simulink model "EffectuatorIntegratedWithDemonstrator"  (R2020a)
settings: Solver=FixedStepDiscrete  StartTime=0.0  StopTime=inf  FixedStep=Ts  RelTol=1e-3
InitFcn:
  | %% Verwende vordefinierte Setpoints (Kreis mit Z-Komponente)
  | 
  | % Config
  | numCircles = 3;
  | scale=6;
  | %Versuch symmetrische Setpunkte zu setzen
  | pointsPerCircle =scale*(4+3*numCircles)+2;
  | 
  | r = 50;
  | m_x = r;
  | m_y = r;
  | 
  | % //
  | s = linspace(0,2*pi,pointsPerCircle);
  | 
  | setPoints_x = [];
  | setPoints_y = [];
  | 
  | for ii=1:numCircles
  | 
  | setPoints_x = [setPoints_x (-cos(s(1:floor(pointsPerCircle / 2))).*r + m_x + 2*r*(ii-1))]; %#ok<AGROW>
  | setPoints_y = [setPoints_y (sin(s).*r+m_y)]; %#ok<AGROW>pointsPerCircle / 2
  | 
  | end
  | 
  | setPoints_x = [setPoints_x flip(setPoints_x(1:end))];
  | 
  | % Loeschen doppelter y-Werte (Kreisuebergang)
  | setPoints_x(pointsPerCircle .* [1:numCircles]) = [];
  | setPoints_y(pointsPerCircle .* [1:numCircles]) = [];
  | 
  | % setPoints_x= [linspace(0,setPoints_x(19),19) setPoints_x(20:end)];
  | % setPoints_y= [linspace(0,setPoints_y(19),19) setPoints_y(20:end)];
  | 
  | % Array Elemente verschieben
  | % setPoints_x = circshift(setPoints_x,-pointsPerCircle/4,2);
  | % setPoints_y = circshift(setPoints_y,-pointsPerCircle/4,2);
  | 
  | z = zeros(1,size(setPoints_x,2));
  | z_x = -5:5;
  | z_y = -z_x.^2 + 25;
  | z_idx = 90;
  | z_idx2 = 210;
  | z(z_idx:z_idx+length(z_x)-1) = z_y;
  | z(z_idx2:z_idx2+length(z_x)-1) = z_y;
  | % z = [z_y z];
  | setPoints_z = z;
  | 
  | % setPoints_x = [zeros(1,length(z_y)) setPoints_x];
  | % setPoints_y = [setPoints_y(1,1)*ones(1,length(z_y)) setPoints_y];
  | 
  | % Umrechnung der Einheiten für Demonstrator
  | % setPoints_x = setPoints_x ./ 1000;
  | % setPoints_y = setPoints_y ./ 1000;
  | % setPoints_z = setPoints_z ./ 1000;
  | 
  | 
  | %{
  | plot(setPoints_x,setPoints_y);
  | fig = figure;
  | ... (+13 lines)
StartFcn:
  | close all;
model workspace (MAT data in the model file):
  MvmtPerfEval_collectVal : Simulink.Parameter (value not decoded)
  MvmtPerfEval_sendOwnVal : Simulink.Parameter (value not decoded)
  PerfEval_numTicks_enable : Simulink.Parameter (value not decoded)
  Segmentregler_I_Gain : Simulink.Parameter (value not decoded)
  Segmentregler_P_Gain : Simulink.Parameter (value not decoded)
  Segmentregler_minVel_enable : Simulink.Parameter (value not decoded)
  Segmentregler_numTicks_enable : Simulink.Parameter (value not decoded)
  Ts : Simulink.Parameter (value not decoded)
  maxPos_x : Simulink.Parameter (value not decoded)
  maxPos_y : Simulink.Parameter (value not decoded)
  maxPos_z : Simulink.Parameter (value not decoded)
  maxVectorLengths : Simulink.Parameter (value not decoded)
  minAllowedVelSaturation : Simulink.Parameter (value not decoded)
  numAxes : Simulink.Parameter (value not decoded)
symbols that are objects in the model workspace (value not decoded): maxPos_x, maxPos_y, maxPos_z, minAllowedVelSaturation, MvmtPerfEval_collectVal, MvmtPerfEval_sendOwnVal, numAxes, PerfEval_numTicks_enable, Segmentregler_I_Gain, Segmentregler_minVel_enable, Segmentregler_numTicks_enable, Segmentregler_P_Gain, Ts
undefined symbols (not defined in the file or in its folder): DiscIntNeverNeededParam, VelOverride
libraries: simulink x20, vrlib x5, sldrtlib x2, xpcrtudplib x2, dspnetwork x2, ptplib x1, etargetslib x1, xpcutilitieslib x1
(part 5 of 5)

== stateflow chart EffectuatorIntegratedWithDemonstrator/MASTER ==
  state funcs [group]
  state Dispatcher [parallel]
    settings: executionOrder=1
    state Idle
    state Registriere_Achse
      entry: num_registeredAxes = ...
      num_registeredAxes + 1;
    state Erhalte_Koordinationsvektor
      entry:
      num_collectedCVectors = ...
      num_collectedCVectors + 1;
      cVectors = [cVectors; cVector_exchange];
      FLAG_canSend_cVector = 1;
    state Distribute_Coordination_Info
      entry:
      FLAG_cVectors_complete = 1;
    state Registriere_Achsen_bereit
      entry:
      num_readyAxes = num_readyAxes + 1;
      if(num_readyAxes == num_registeredAxes)
      FLAG_allAxesReady = 1;
      messageToEffectuator=2;
      end
    state DONE
      entry:
      num_doneAxes = num_doneAxes + 1;
      if num_doneAxes == num_registeredAxes
      FLAG_stopSim = 1;
      end
    state Movement_Performance_Evaluation
      entry:
      segmentDone=segmentDone+1;
      if (segmentDone==num_registeredAxes)
      canStartNewSegment=1;
      segmentDone=0;
      else
      canStartNewSegment=0;
      end
      while receive(MvmtPerfCoeff)
      if MvmtPerfCoeff.data > MvmtPerf
      MvmtPerf = MvmtPerfCoeff.data;
      end
      if MvmtPerfCoeff.data == -1
      MvmtPerf = 1;
      end
      discard(MvmtPerfCoeff);
      end
    (default) -> Idle
    Idle -> Registriere_Achse [order 1] : registerAxis
    Registriere_Achse -> Idle
    Idle -> Erhalte_Koordinationsvektor [order 2] : cVector_sent
    Erhalte_Koordinationsvektor -> Idle
    Idle -> Distribute_Coordination_Info [order 3] : [num_collectedCVectors==...
        | num_registeredAxes && ...
        | FLAG_cVectors_complete == 0]
    Distribute_Coordination_Info -> Idle
    Idle -> Registriere_Achsen_bereit [order 4] : axis_ready
    Registriere_Achsen_bereit -> Idle
    Idle -> Dispatcher.DONE [order 5] : axis_done
    Dispatcher.DONE -> Idle
    Idle -> Movement_Performance_Evaluation [order 6] : MvmtPerfCoeff
    Movement_Performance_Evaluation -> Idle
  state Axis_X [parallel]
    settings: executionOrder=2
    state Start_Idle
      entry:
      registerAxis.data = true;
      send(registerAxis)
    state Hermite_Interpolation
      entry:
      if FLAG_doAkima == 1
      iP = funcs.DS_hermIntp(setP,setP_dist);
      else
      iP = setP;
      end
    state Koordinationsvektor
      entry:
      cVector_init = funcs.DS_gen_Cvector_init...
      (iP,PAR_isAxis,PAR_maxVel);
    state Koordinationsvektor_austauschen
      during:
      if FLAG_canSend_cVector == 1
      cVector_exchange = cVector_init;
      FLAG_canSend_cVector = 0;
      send(cVector_sent);
      axisHasSentCVector = 1;
      end
      Axis_X.Koordinationsvektor_austauschen -> Axis_X.Koordinationsvektor_austauschen [order 1]
    state Wait_for_cVectors
    state Find_Consensus
      entry: execVec = funcs.DS_find_Consensus(iP,cVectors,...
      PAR_execIteratorStepSize,PAR_isAxis);
      send(axis_ready);
    state Start_run
      entry:
      RUN_idx = 0;
      RUN_startPos(1,PAR_isAxis) = setP(PAR_isAxis,1);
      RUN_num_steps = size(execVec,2);
      state Send_command
        entry:
        RUN_idx = RUN_idx + 1;
        currCVector = cVectors(:,RUN_idx)' ./ VelOverride';
        currCVal = max(currCVector);
        currOverrideAdaptationFactor = execVec(3,RUN_idx) / currCVal; %individueller neuer Override Faktor für diese Achse
        currStepTimeLength = execVec(3,RUN_idx) / currOverrideAdaptationFactor;
        RUN_pos(1,PAR_isAxis) = execVec(1,RUN_idx);
        RUN_vel(1,PAR_isAxis) = execVec(2,RUN_idx) * currOverrideAdaptationFactor;
        MvmtPerf_accumulatedLagTime = MvmtPerf_accumulatedLagTime + (currStepTimeLength - execVec(3,RUN_idx));
        RUN_time(1,PAR_isAxis) = execVec(4,RUN_idx) + MvmtPerf_accumulatedLagTime; %wird nicht benutzt
        RUN_maxVel(1,PAR_isAxis) = PAR_maxVel;
        RUN_MvmtPerfFeedback(1,PAR_isAxis) = 0; %wird zZt nicht benutzt
      state execute_movement
        state idle
          entry:
          MvmtPerfCoeff.data = -1;
          send(MvmtPerfCoeff);
        state getOwnPerfCoeff [commented out]
          entry:
          MvmtPerfCoeff.data = GET_perfIndicator(PAR_isAxis);
          send(MvmtPerfCoeff);
        state getMutualPerformance [commented out]
          entry:
          MvmtPerf_accumulatedLagTime = MvmtPerf_accumulatedLagTime + (MvmtPerf-1) * currStepTimeLength;
          RUN_MvmtPerfFeedback(1,PAR_isAxis) = (MvmtPerf-1) * currStepTimeLength;
          RUN_vel(1,PAR_isAxis) = execVec(2,RUN_idx) / MvmtPerf;
          currStepTimeLength = currStepTimeLength * MvmtPerf;
        (default) -> Axis_X.Start_run.execute_movement.idle
        Axis_X.Start_run.execute_movement.idle -> Axis_X.Start_run.execute_movement.getOwnPerfCoeff [commented out] : after(currStepTimeLength * MvmtPerfEval_sendOwnVal,sec)
        Axis_X.Start_run.execute_movement.getOwnPerfCoeff -> Axis_X.Start_run.execute_movement.getMutualPerformance [commented out] : after(currStepTimeLength * (MvmtPerfEval_collectVal - MvmtPerfEval_sendOwnVal),sec)
      (default) -> Axis_X.Start_run.Send_command
      (junction 638) -> Axis_X.Start_run.Send_command [order 2]
      Axis_X.Start_run.Send_command -> Axis_X.Start_run.execute_movement
      (junction 1327) -> (junction 638) : [index<=EffSegment(1)]
      Axis_X.Start_run.execute_movement -> (junction 1327) : after(currStepTimeLength,sec)
    state DONE
      entry:
      send(axis_done);
    (default) -> Axis_X.Start_Idle
    Axis_X.Start_Idle -> Axis_X.Hermite_Interpolation
    Axis_X.Hermite_Interpolation -> Axis_X.Koordinationsvektor
    Axis_X.Koordinationsvektor -> Axis_X.Koordinationsvektor_austauschen
    Axis_X.Koordinationsvektor_austauschen -> Axis_X.Wait_for_cVectors [order 1] : [axisHasSentCVector == 1]
    Axis_X.Wait_for_cVectors -> Axis_X.Find_Consensus : [FLAG_cVectors_complete == 1]
    Axis_X.Find_Consensus -> Axis_X.Start_run : [FLAG_allAxesReady == 1]
    (junction 638) -> Axis_X.DONE [order 1] : [RUN_idx == RUN_num_steps]
  state Axis_Y [parallel]
    settings: executionOrder=3
    state Start_Idle
      entry:
      registerAxis.data = true;
      send(registerAxis)
    state Hermite_Interpolation
      entry:
      if FLAG_doAkima == 1
      iP = funcs.DS_hermIntp(setP,setP_dist);
      else
      iP = setP;
      end
    state Koordinationsvektor
      entry:
      cVector_init = funcs.DS_gen_Cvector_init...
      (iP,PAR_isAxis,PAR_maxVel);
    state Koordinationsvektor_austauschen
      during:
      if FLAG_canSend_cVector == 1
      cVector_exchange = cVector_init;
      FLAG_canSend_cVector = 0;
      send(cVector_sent);
      axisHasSentCVector = 1;
      end
      Axis_Y.Koordinationsvektor_austauschen -> Axis_Y.Koordinationsvektor_austauschen [order 1]
    state Wait_for_cVectors
    state Find_Consensus
      entry: execVec = funcs.DS_find_Consensus(iP,cVectors,...
      PAR_execIteratorStepSize,PAR_isAxis);
      send(axis_ready);
    state Start_run
      entry:
      RUN_idx = 0;
      RUN_startPos(1,PAR_isAxis) = setP(PAR_isAxis,1);
      RUN_num_steps = size(execVec,2);
      state Send_command
        entry:
        RUN_idx = RUN_idx + 1;
        currCVector = cVectors(:,RUN_idx)' ./ VelOverride';
        currCVal = max(currCVector);
        currOverrideAdaptationFactor = execVec(3,RUN_idx) / currCVal; %individueller neuer Override Faktor für diese Achse
        currStepTimeLength = execVec(3,RUN_idx) / currOverrideAdaptationFactor;
        RUN_pos(1,PAR_isAxis) = execVec(1,RUN_idx);
        RUN_vel(1,PAR_isAxis) = execVec(2,RUN_idx) * currOverrideAdaptationFactor;
        MvmtPerf_accumulatedLagTime = MvmtPerf_accumulatedLagTime + (currStepTimeLength - execVec(3,RUN_idx));
        RUN_time(1,PAR_isAxis) = execVec(4,RUN_idx) + MvmtPerf_accumulatedLagTime; %wird nicht benutzt
        RUN_maxVel(1,PAR_isAxis) = PAR_maxVel;
        RUN_MvmtPerfFeedback(1,PAR_isAxis) = 0; %wird zZt nicht benutzt
      state execute_movement
        state idle
          entry:
          MvmtPerfCoeff.data = -1;
          send(MvmtPerfCoeff);
          index=RUN_idx;
        state getOwnPerfCoeff [commented out]
          entry:
          MvmtPerfCoeff.data = GET_perfIndicator(PAR_isAxis);
          send(MvmtPerfCoeff);
        state getMutualPerformance [commented out]
          entry:
          MvmtPerf_accumulatedLagTime = MvmtPerf_accumulatedLagTime + (MvmtPerf-1) * currStepTimeLength;
          RUN_MvmtPerfFeedback(1,PAR_isAxis) = (MvmtPerf-1) * currStepTimeLength;
          RUN_vel(1,PAR_isAxis) = execVec(2,RUN_idx) / MvmtPerf;
          currStepTimeLength = currStepTimeLength * MvmtPerf;
        (default) -> Axis_Y.Start_run.execute_movement.idle
        Axis_Y.Start_run.execute_movement.idle -> Axis_Y.Start_run.execute_movement.getOwnPerfCoeff [commented out] : after(currStepTimeLength * MvmtPerfEval_sendOwnVal,sec)
        Axis_Y.Start_run.execute_movement.getOwnPerfCoeff -> Axis_Y.Start_run.execute_movement.getMutualPerformance [commented out] : after(currStepTimeLength * (MvmtPerfEval_collectVal - MvmtPerfEval_sendOwnVal),sec)
      (default) -> Axis_Y.Start_run.Send_command
      (junction 1151) -> Axis_Y.Start_run.Send_command [order 2]
      Axis_Y.Start_run.Send_command -> Axis_Y.Start_run.execute_movement
      (junction 1322) -> (junction 1151) : [index<=EffSegment(1)]
      Axis_Y.Start_run.execute_movement -> (junction 1322) : after(currStepTimeLength,sec)
    state DONE
      entry:
      send(axis_done);
    (default) -> Axis_Y.Start_Idle
    Axis_Y.Start_Idle -> Axis_Y.Hermite_Interpolation
    Axis_Y.Hermite_Interpolation -> Axis_Y.Koordinationsvektor
    Axis_Y.Koordinationsvektor -> Axis_Y.Koordinationsvektor_austauschen
    Axis_Y.Koordinationsvektor_austauschen -> Axis_Y.Wait_for_cVectors [order 1] : [axisHasSentCVector == 1]
    Axis_Y.Wait_for_cVectors -> Axis_Y.Find_Consensus : [FLAG_cVectors_complete == 1]
    Axis_Y.Find_Consensus -> Axis_Y.Start_run : [FLAG_allAxesReady == 1]
    (junction 1151) -> Axis_Y.DONE [order 1] : [RUN_idx == RUN_num_steps]
  state Axis_Z [parallel]
    settings: executionOrder=4
    state Start_Idle
      entry:
      registerAxis.data = true;
      send(registerAxis)
    state Hermite_Interpolation
      entry:
      if FLAG_doAkima == 1
      iP = funcs.DS_hermIntp(setP,setP_dist);
      else
      iP = setP;
      end
    state Koordinationsvektor
      entry:
      cVector_init = funcs.DS_gen_Cvector_init...
      (iP,PAR_isAxis,PAR_maxVel);
    state Koordinationsvektor_austauschen
      during:
      if FLAG_canSend_cVector == 1
      cVector_exchange = cVector_init;
      FLAG_canSend_cVector = 0;
      send(cVector_sent);
      axisHasSentCVector = 1;
      end
      Axis_Z.Koordinationsvektor_austauschen -> Axis_Z.Koordinationsvektor_austauschen [order 1]
    state Wait_for_cVectors
    state Find_Consensus
      entry: execVec = funcs.DS_find_Consensus(iP,cVectors,...
      PAR_execIteratorStepSize,PAR_isAxis);
      send(axis_ready);
    state Start_run
      entry:
      RUN_idx = 0;
      RUN_startPos(1,PAR_isAxis) = setP(PAR_isAxis,1);
      RUN_num_steps = size(execVec,2);
      state Send_command
        entry:
        RUN_idx = RUN_idx + 1;
        currCVector = cVectors(:,RUN_idx)' ./ VelOverride';
        currCVal = max(currCVector);
        currOverrideAdaptationFactor = execVec(3,RUN_idx) / currCVal; %individueller neuer Override Faktor für diese Achse
        currStepTimeLength = execVec(3,RUN_idx) / currOverrideAdaptationFactor;
        RUN_pos(1,PAR_isAxis) = execVec(1,RUN_idx);
        RUN_vel(1,PAR_isAxis) = execVec(2,RUN_idx) * currOverrideAdaptationFactor;
        MvmtPerf_accumulatedLagTime = MvmtPerf_accumulatedLagTime + (currStepTimeLength - execVec(3,RUN_idx));
        RUN_time(1,PAR_isAxis) = execVec(4,RUN_idx) + MvmtPerf_accumulatedLagTime; %wird nicht benutzt
        RUN_maxVel(1,PAR_isAxis) = PAR_maxVel;
        RUN_MvmtPerfFeedback(1,PAR_isAxis) = 0; %wird zZt nicht benutzt
      state execute_movement
        state idle
          entry:
          MvmtPerfCoeff.data = -1;
          send(MvmtPerfCoeff);
        state getOwnPerfCoeff [commented out]
          entry:
          MvmtPerfCoeff.data = GET_perfIndicator(PAR_isAxis);
          send(MvmtPerfCoeff);
        state getMutualPerformance [commented out]
          entry:
          MvmtPerf_accumulatedLagTime = MvmtPerf_accumulatedLagTime + (MvmtPerf-1) * currStepTimeLength;
          RUN_MvmtPerfFeedback(1,PAR_isAxis) = (MvmtPerf-1) * currStepTimeLength;
          RUN_vel(1,PAR_isAxis) = execVec(2,RUN_idx) / MvmtPerf;
          currStepTimeLength = currStepTimeLength * MvmtPerf;
        (default) -> Axis_Z.Start_run.execute_movement.idle
        Axis_Z.Start_run.execute_movement.idle -> Axis_Z.Start_run.execute_movement.getOwnPerfCoeff [commented out] : after(currStepTimeLength * MvmtPerfEval_sendOwnVal,sec)
        Axis_Z.Start_run.execute_movement.getOwnPerfCoeff -> Axis_Z.Start_run.execute_movement.getMutualPerformance [commented out] : after(currStepTimeLength * (MvmtPerfEval_collectVal - MvmtPerfEval_sendOwnVal),sec)
      (default) -> Axis_Z.Start_run.Send_command
      (junction 1195) -> Axis_Z.Start_run.Send_command [order 2]
      Axis_Z.Start_run.Send_command -> Axis_Z.Start_run.execute_movement
      (junction 1320) -> (junction 1195) : [index<=EffSegment(1)]
      Axis_Z.Start_run.execute_movement -> (junction 1320) : after(currStepTimeLength,sec)
    state DONE
      entry:
      send(axis_done);
    (default) -> Axis_Z.Start_Idle
    Axis_Z.Start_Idle -> Axis_Z.Hermite_Interpolation
    Axis_Z.Hermite_Interpolation -> Axis_Z.Koordinationsvektor
    Axis_Z.Koordinationsvektor -> Axis_Z.Koordinationsvektor_austauschen
    Axis_Z.Koordinationsvektor_austauschen -> Axis_Z.Wait_for_cVectors [order 1] : [axisHasSentCVector == 1]
    Axis_Z.Wait_for_cVectors -> Axis_Z.Find_Consensus : [FLAG_cVectors_complete == 1]
    Axis_Z.Find_Consensus -> Axis_Z.Start_run : [FLAG_allAxesReady == 1]
    (junction 1195) -> Axis_Z.DONE [order 1] : [RUN_idx == RUN_num_steps]
  state Axis_X2_Effectuator [parallel]
    settings: executionOrder=5
    state Start_Idle
      entry:
      registerAxis.data = true;
      send(registerAxis)
    state Hermite_Interpolation
      entry:
      if FLAG_doAkima == 1
      iP = funcs.DS_hermIntp(setP,setP_dist);
      else
      iP = setP;
      end
    state Koordinationsvektor
      entry:
      cVector_init = Axis_X2_koordVector;
    state Koordinationsvektor_austauschen
      during:
      if FLAG_canSend_cVector == 1
      cVector_exchange = cVector_init;
      FLAG_canSend_cVector = 0;
      send(cVector_sent);
      axisHasSentCVector = 1;
      messageToEffectuator=1;
      end
      Axis_X2_Effectuator.Koordinationsvektor_austauschen -> Axis_X2_Effectuator.Koordinationsvektor_austauschen [commented out]
    state Wait_for_cVectors
    state Find_Consensus
      entry: execVec =Axis_X2_consusVector;
      send(axis_ready);
    state execute_movement1 [commented out]
      state idle [commented out]
        entry:
        MvmtPerfCoeff.data = -1;
        send(MvmtPerfCoeff);
      state getOwnPerfCoeff [commented out]
        entry:
        MvmtPerfCoeff.data = GET_perfIndicator(PAR_isAxis);
        send(MvmtPerfCoeff);
      state getMutualPerformance [commented out]
        entry:
        MvmtPerf_accumulatedLagTime = MvmtPerf_accumulatedLagTime + (MvmtPerf-1) * currStepTimeLength;
        RUN_MvmtPerfFeedback(1,PAR_isAxis) = (MvmtPerf-1) * currStepTimeLength;
        RUN_vel(1,PAR_isAxis) = execVec(2,RUN_idx) / MvmtPerf;
        currStepTimeLength = currStepTimeLength * MvmtPerf;
      (default) -> Axis_X2_Effectuator.execute_movement1.idle [commented out]
      Axis_X2_Effectuator.execute_movement1.idle -> Axis_X2_Effectuator.execute_movement1.getOwnPerfCoeff [commented out] : after(currStepTimeLength * MvmtPerfEval_sendOwnVal,sec)
      Axis_X2_Effectuator.execute_movement1.getOwnPerfCoeff -> Axis_X2_Effectuator.execute_movement1.getMutualPerformance [commented out] : after(currStepTimeLength * (MvmtPerfEval_collectVal - MvmtPerfEval_sendOwnVal),sec)
    state Start_run [commented out]
      entry:
      RUN_idx = 0;
      RUN_startPos(1,PAR_isAxis) = setP(PAR_isAxis,1);
      RUN_num_steps = size(execVec,2);
      state Send_command [commented out]
        entry:
        RUN_idx = RUN_idx + 1;
        currCVector = cVectors(:,RUN_idx)' ./ VelOverride';
        currCVal = max(currCVector);
        currOverrideAdaptationFactor = execVec(3,RUN_idx) / currCVal; %individueller neuer Override Faktor für diese Achse
        currStepTimeLength = execVec(3,RUN_idx) / currOverrideAdaptationFactor;
        RUN_pos(1,PAR_isAxis) = execVec(1,RUN_idx);
        RUN_vel(1,PAR_isAxis) = execVec(2,RUN_idx) * currOverrideAdaptationFactor;
        MvmtPerf_accumulatedLagTime = MvmtPerf_accumulatedLagTime + (currStepTimeLength - execVec(3,RUN_idx));
        RUN_time(1,PAR_isAxis) = execVec(4,RUN_idx) + MvmtPerf_accumulatedLagTime; %wird nicht benutzt
        RUN_maxVel(1,PAR_isAxis) = PAR_maxVel;
        RUN_MvmtPerfFeedback(1,PAR_isAxis) = 0; %wird zZt nicht benutzt
      state execute_movement [commented out]
        state idle [commented out]
          entry:
          MvmtPerfCoeff.data = -1;
          send(MvmtPerfCoeff);
        state getOwnPerfCoeff [commented out]
          entry:
          MvmtPerfCoeff.data = GET_perfIndicator(PAR_isAxis);
          send(MvmtPerfCoeff);
        state getMutualPerformance [commented out]
          entry:
          MvmtPerf_accumulatedLagTime = MvmtPerf_accumulatedLagTime + (MvmtPerf-1) * currStepTimeLength;
          RUN_MvmtPerfFeedback(1,PAR_isAxis) = (MvmtPerf-1) * currStepTimeLength;
          RUN_vel(1,PAR_isAxis) = execVec(2,RUN_idx) / MvmtPerf;
          currStepTimeLength = currStepTimeLength * MvmtPerf;
        (default) -> Axis_X2_Effectuator.Start_run.execute_movement.idle [commented out]
        Axis_X2_Effectuator.Start_run.execute_movement.idle -> Axis_X2_Effectuator.Start_run.execute_movement.getOwnPerfCoeff [commented out] : after(currStepTimeLength * MvmtPerfEval_sendOwnVal,sec)
        Axis_X2_Effectuator.Start_run.execute_movement.getOwnPerfCoeff -> Axis_X2_Effectuator.Start_run.execute_movement.getMutualPerformance [commented out] : after(currStepTimeLength * (MvmtPerfEval_collectVal - MvmtPerfEval_sendOwnVal),sec)
      (default) -> Axis_X2_Effectuator.Start_run.Send_command [commented out]
      (junction 1244) -> Axis_X2_Effectuator.Start_run.Send_command [commented out]
      Axis_X2_Effectuator.Start_run.Send_command -> Axis_X2_Effectuator.Start_run.execute_movement [commented out]
      Axis_X2_Effectuator.Start_run.execute_movement -> (junction 1244) [commented out] : after(currStepTimeLength,sec)
    state DONE
      entry:
      send(axis_done);
    (default) -> Axis_X2_Effectuator.Start_Idle
    Axis_X2_Effectuator.Start_Idle -> Axis_X2_Effectuator.Hermite_Interpolation
    Axis_X2_Effectuator.Hermite_Interpolation -> Axis_X2_Effectuator.Koordinationsvektor : [messageFromEffectuator==1]
    Axis_X2_Effectuator.Koordinationsvektor -> Axis_X2_Effectuator.Koordinationsvektor_austauschen
    Axis_X2_Effectuator.Koordinationsvektor_austauschen -> Axis_X2_Effectuator.Wait_for_cVectors : [axisHasSentCVector == 1]
    Axis_X2_Effectuator.Wait_for_cVectors -> Axis_X2_Effectuator.Find_Consensus : [FLAG_cVectors_complete == 1&&messageFromEffectuator==2]
    Axis_X2_Effectuator.Find_Consensus -> Axis_X2_Effectuator.DONE : [messageFromEffectuator==4]
  data: inp_data function_input; iPoints function_output; iP_dist function_input; inp_data function_input; whichAxis function_input; cV_init function_output; maxV function_input; iPoints function_input; cVec function_input; execVec function_output; iteratorStep function_input; whichAxis function_input; inp_data function_input; iPoints function_output; iP_dist function_input; num_registeredAxes local =0; num_collectedCVectors local =0; iP local size=[numAxes maxVectorLengths]; cVector_init local size=[1 maxVectorLengths]; PAR_isAxis constant double =1; PAR_maxVel constant double =10; axisHasSentCVector local =0; execVec local size=[4 maxVectorLengths] =1; RUN_idx local double size=1 =0; currStepTimeLength local =0; RUN_num_steps local =0; MvmtPerf_accumulatedLagTime local =0; currCVector local size=[1 numAxes] =zeros(1,numAxes); currCVal local =0; currOverrideAdaptationFactor local =1; isUDP_Agent local =0; iP local size=[numAxes maxVectorLengths]; cVector_init local size=[1 maxVectorLengths]; PAR_isAxis constant double =2; PAR_maxVel constant double =5; axisHasSentCVector local =0; execVec local size=[4 maxVectorLengths] =1; RUN_idx local size=1 =0; currStepTimeLength local =0; RUN_num_steps local =0; MvmtPerf_accumulatedLagTime local =0; currCVector local size=[1 numAxes] =zeros(1,numAxes); currCVal local =0; currOverrideAdaptationFactor local =1; isUDP_Agent local =0; iP local size=[numAxes maxVectorLengths]; cVector_init local size=[1 maxVectorLengths]; PAR_isAxis constant double =3; PAR_maxVel constant double =2; axisHasSentCVector local =0; execVec local size=[4 maxVectorLengths] =1; RUN_idx local size=1 =0; currStepTimeLength local =0; RUN_num_steps local =0; MvmtPerf_accumulatedLagTime local =0; currCVector local size=[1 numAxes] =zeros(1,numAxes); currCVal local =0; currOverrideAdaptationFactor local =1; isUDP_Agent local =0; iP local size=[numAxes maxVectorLengths]; cVector_init local size=[1 maxVectorLengths]; PAR_isAxis constant double =4; PAR_maxVel constant double =5; axisHasSentCVector local =0; execVec local size=[4 maxVectorLengths] =1; RUN_idx local size=1 =0; currStepTimeLength local =0; RUN_num_steps local =0; MvmtPerf_accumulatedLagTime local =0; currCVector local size=[1 numAxes] =zeros(1,numAxes); currCVal local =0; currOverrideAdaptationFactor local =1; isUDP_Agent local =1; setP input; setP_dist input; registerAxis local; FLAG_canSend_cVector local =1; cVector_exchange local size=[1 maxVectorLengths]; cVector_sent local =1; FLAG_cVectors_complete local =0; PAR_execIteratorStepSize constant double =1; axis_ready local =0; num_readyAxes local =0; FLAG_allAxesReady local =0; FLAG_doAkima local =0; axis_done local =0; FLAG_stopSim output =0; RUN_maxVel output size=[1 numAxes] =zeros(1,numAxes); RUN_pos output size=[1 numAxes] =zeros(1,numAxes); RUN_startPos output size=[1 numAxes] =zeros(1,numAxes); RUN_time output size=[1 numAxes] =zeros(1,numAxes); RUN_vel output size=[1 numAxes] =zeros(1,numAxes); MvmtPerfEval_sendOwnVal parameter; GET_perfIndicator data_store_memory; MvmtPerfCoeff local =1; MvmtPerf local =1; RUN_MvmtPerfFeedback output size=[1 numAxes] =zeros(1,numAxes); MvmtPerfEval_collectVal parameter; VelOverride data_store_memory; cVectors output size=[numAxes maxVectorLengths] =0; Axis_X2_koordVector input; Axis_X2_consusVector input; messageFromEffectuator input int32 [..int32(0)]; messageToEffectuator output int32 =int32(0); num_doneAxes output =0; EffSegment input; segmentDone local =0; canStartNewSegment output =0; index output
  events: event local FUNCTION_CALL_EVENT
  function iPoints = DS_hermIntp(inp_data,iP_dist):
    | function iPoints = DS_hermIntp(inp_data,iP_dist)
    |  
    | 
    | euklid_abstand = vecnorm(diff(inp_data,1,2));
    | 
    | laufparam = cumsum(euklid_abstand);
    | laufparam = laufparam / max(laufparam);
    | laufparam = [0 laufparam];
    | 
    | 
    | anzahl_stuetzpunkte = 150;
    | anzahl_dim = size(inp_data,1);
    | iPoints = zeros(anzahl_dim,anzahl_stuetzpunkte);
    | 
    | for i=1:anzahl_dim
    |    
    |     iPoints(i,:) = pchip(laufparam,inp_data(i,:),linspace(0,1,anzahl_stuetzpunkte));
    |     
    | end
    | 
    | end
  function cV_init = DS_gen_Cvector_init(inp_data,whichAxis,maxV):
    | function cV_init = DS_gen_Cvector_init(inp_data,whichAxis,maxV)
    | 
    | safety_margin = 0.2; % max. Geschwindigkeit wird auf 80% der eigentlichen Fähigkeit der Achse festgelegt
    | 
    | wegdaten_raw = inp_data(whichAxis,:);
    | 
    | streckensegmente_raw = diff(wegdaten_raw);
    | 
    | 
    | zeitsegmente_raw = streckensegmente_raw ./ (maxV * (1 - safety_margin));
    | 
    | 
    | cV_init = abs(zeitsegmente_raw);
    | 
    | end
  function execVec = DS_find_Consensus(iPoints,cVec,iteratorStep,whichAxis):
    | function execVec = DS_find_Consensus(iPoints,cVec,iteratorStep,whichAxis)
    | 
    | cVector = max(cVec);
    | 
    | if(iteratorStep > 1)
    |    
    |     if(mod(size(iPoints,2)-1,iteratorStep) == 0)
    |         
    |         array_size = (size(iPoints,2) - 1) / iteratorStep;
    |         iPoints_relevant = zeros(1,array_size);
    |         
    |     else
    |        
    |         array_size = floor((size(iPoints,2) - 1) / iteratorStep) + 1;
    |         iPoints_relevant = zeros(1,array_size);
    |         
    |     end
    |     
    |     
    |     iPoints_relevant = iPoints(whichAxis,1:iteratorStep:end);
    |     
    |     % Neue Zeitabschnitte berechnen
    |     for ii=1:array_size-1
    |        
    |         currIdx = ((ii-1) * iteratorStep) + 1;
    |         zP = cVec(1,currIdx : currIdx + iteratorStep);
    |         
    |         zeitabschnitte = sum(zP);
    |         
    |     end
    | 
    |     
    | else
    |    
    |     iPoints_relevant = iPoints(whichAxis,:);
    | 
    |     
    | end
    | 
    |     wegabschnitte = diff(iPoints_relevant(1,:));
    |     zeitabschnitte = cVector;
    |     absolute_zeitpunkte = cumsum(zeitabschnitte);
    |     
    |     geschwindigkeiten = abs(wegabschnitte ./ zeitabschnitte);
    |     
    |     execVec = [iPoints_relevant(2:end);...
    |         geschwindigkeiten;...
    |         zeitabschnitte;...
    |         absolute_zeitpunkte];
    | 
    | 
    | 
    | end
  function iPoints = DS_hermIntp_old(inp_data,iP_dist):
    | function iPoints = DS_hermIntp_old(inp_data,iP_dist)
    |  
    | x = inp_data(1,:);
    | y = inp_data(2,:);
    | 
    | x_zwischenpunkte = (x(1):iP_dist:x(end));
    | 
    | y_interpoliert = pchip(x,y,x_zwischenpunkte);
    | 
    | iPoints = [x_zwischenpunkte; y_interpoliert];
    | 
    | 
    | end

== stateflow chart EffectuatorIntegratedWithDemonstrator/PosTracer_v2 ==
  state Create_Plot
    entry:
    startPos = DS_createTracePlot(numAxes);
  state Fetch_Positions
    entry:
    for ii=1:size(GET_istPos,1)
    switch ii
    case 1
    pos_x = GET_istPos(ii);
    case 2
    pos_y = GET_istPos(ii);
    case 3
    pos_z = GET_istPos(ii);
    case 4
    pos_x2 = EffsegmentData(2)/10000;
    end
    end
  state Update_Plot
    entry:
    if numAxes == 2
    DS_updateTracePlot(numAxes,pos_x+startPos(1,1),pos_y+startPos(1,2),0,false);
    elseif numAxes == 3
    DS_updateTracePlot(numAxes,pos_x+startPos(1,1),pos_y+startPos(1,2),...
    pos_z+startPos(1,3),true);
    elseif (numAxes == 4 )
    if (num_doneAxes<3)
    DS_updateTracePlot(numAxes,pos_x+startPos(1,1),pos_y+startPos(1,2),...
    pos_z+startPos(1,3),true);
    end
    DS_updateTraceEff(numAxes,pos_x2,EffsegmentData(1),true)
    end
  (default) -> Create_Plot
  Create_Plot -> Fetch_Positions
  Fetch_Positions -> Update_Plot
  Update_Plot -> Fetch_Positions : after(35,tick)
  data: numAx function_input; sPos function_output; numAx function_input; pos1 function_input; pos2 function_input; pos3 function_input; drawLine function_input; numAx function_input; pos4 function_input; index function_input; drawLine function_input; numAxes parameter; pos_x local =0; pos_y local =0; GET_istPos data_store_memory; pos_z local =0; startPos local size=[1 numAxes] =zeros(1,numAxes); ii local; pos_x2 local =0; num_doneAxes input; EffsegmentData input
  function sPos  = DS_createTracePlot(numAx):
    | function sPos  = DS_createTracePlot(numAx)
    | 
    | coder.extrinsic('evalin');
    | coder.extrinsic('setappdata');
    | 
    | setP = evalin('base','setP_mat');
    | 
    | sPos = zeros(1,numAx);
    | if(numAx == 4)
    |     fig = figure;
    |     ax = axes;
    |         
    |     [~,dim2,~] = size(setP);
    |     plot3(ax,setP(1,1:dim2),setP(2,1:dim2),setP(3,1:dim2));
    |     
    |     set(fig,'Tag','TraceFig');
    |     set(ax,'Tag','TraceAxes');
    |     set(ax,'NextPlot','add');
    |     set(ax,'YDir','reverse');
    |     set(ax,'ZDir','reverse');
    |     
    |     sPos(1,1) = setP(1,1);
    |     sPos(1,2) = setP(2,1);
    |     sPos(1,3) = setP(3,1);
    |     
    |     traceLine = plot3(ax,[setP(1,1) setP(1,1)],[setP(2,1) setP(2,1)],[setP(3,1) setP(3,1)],'Color',[0 0 1],'LineWidth',1);
    |     setappdata(ax,'traceLine',traceLine);
    |     %    Effectuator axis   
    | 
    | [~,dim2,~] = size(setP);
    | sPos(1,4) = setP(1,1);
    | fig2 = figure;
    | ax2 = axes;
    | y = setP(1,1:dim2);
    | set(fig2,'Tag','TraceFig2');
    | set(ax2,'Tag','TraceAxes2');
    | set(ax2,'NextPlot','add');
    | plot(ax2,y)
    | xlabel('Segment')
    | ylabel('Position')
    | hold on
    | p = plot(ax2(1),y(1),'o','MarkerFaceColor',[1 213/255 0]);
    | setappdata(ax2,'traceLine2',p);
    | hold off
    | axis manual
    |  
    | 
    | elseif(numAx == 3)
    |     fig = figure;
    |     ax = axes;
    |         
    |     [~,dim2,~] = size(setP);
    |     plot3(ax,setP(1,1:dim2),setP(2,1:dim2),setP(3,1:dim2));
    |     
    |     set(fig,'Tag','TraceFig');
    |     set(ax,'Tag','TraceAxes');
    |     set(ax,'NextPlot','add');
    |     set(ax,'YDir','reverse');
    |     set(ax,'ZDir','reverse');
    |     
    |     sPos(1,1) = setP(1,1);
    |     sPos(1,2) = setP(2,1);
    |     sPos(1,3) = setP(3,1);
    |     
    |     traceLine = plot3(ax,[setP(1,1) setP(1,1)],[setP(2,1) setP(2,1)],[setP(3,1) setP(3,1)],'Color',[0 0 1],'LineWidth',1);
    |     setappdata(ax,'traceLine',traceLine);
    |     
    | elseif(numAx == 2)
    |     
    |     fig = figure;
    |     ax = axes;
    |         
    |     [~,dim2] = size(setP);
    |     plot(ax,setP(1,1:dim2),setP(2,1:dim2));
    |     
    |     set(fig,'Tag','TraceFig');
    |     set(ax,'Tag','TraceAxes');
    |     set(ax,'NextPlot','add');
    |     
    |     sPos(1,1) = setP(1,1);
    |     sPos(1,2) = setP(2,1);
    |     
    |     traceLine = plot(ax,[setP(1,1) setP(1,1)],[setP(2,1) setP(2,1)],'Color',[0 0 1],'LineWidth',1);
    |     setappdata(ax,'traceLine',traceLine);
    |     
    | end
    | 
    | end
  function DS_updateTracePlot(numAx,pos1,pos2,pos3,drawLine):
    | function DS_updateTracePlot(numAx,pos1,pos2,pos3,drawLine)
    | 
    | coder.extrinsic('delete');
    | coder.extrinsic('scatter');
    | coder.extrinsic('scatter3');
    | coder.extrinsic('getappdata');
    | coder.extrinsic('setappdata');
    | 
    | 
    |     
    |    ax = findobj('Tag','TraceAxes');
    |    punkt = getappdata(ax,'tracePunkt');
    | 
    |    if ~isempty(punkt)
    |     delete(punkt);
    |    end
    | 
    | 
    | 
    | if(numAx == 4)
    |    
    |     punkt = scatter3(ax,pos1,pos2,pos3,'MarkerEdgeColor','r','LineWidth',2);
    |     setappdata(ax,'tracePunkt',punkt);
    |     
    |     if drawLine
    |        
    |         traceLine = getappdata(ax,'traceLine');
    |         
    |         XData = get(traceLine,'XData');
    |         YData = get(traceLine,'YData');
    |         ZData = get(traceLine,'ZData');
    |     
    |         set(traceLine,'XData',[XData pos1]);
    |         set(traceLine,'YData',[YData pos2]);
    |         set(traceLine,'ZData',[ZData pos3]);
    |        
    |            
    |     end
    | elseif(numAx == 3)
    |     
    |     punkt = scatter3(ax,pos1,pos2,pos3,'MarkerEdgeColor','r','LineWidth',2);
    |     setappdata(ax,'tracePunkt',punkt);
    |     
    |     if drawLine
    |         
    |         traceLine = getappdata(ax,'traceLine');
    |         XData = get(traceLine,'XData');
    |         YData = get(traceLine,'YData');
    |         ZData = get(traceLine,'ZData');
    |         
    |         set(traceLine,'XData',[XData pos1]);
    |         set(traceLine,'YData',[YData pos2]);
    |         set(traceLine,'ZData',[ZData pos3]);
    |         
    |     end
    |     
    | elseif(numAx == 2)
    |     
    |     punkt = scatter(ax,pos1,pos2,'MarkerEdgeColor','r','LineWidth',2);
    |     setappdata(ax,'tracePunkt',punkt);
    |     
    |     if drawLine
    |         
    |         traceLine = getappdata(ax,'traceLine');
    |         XData = get(traceLine,'XData');
    |         YData = get(traceLine,'YData');
    |         
    |         set(traceLine,'XData',[XData pos1]);
    |         set(traceLine,'YData',[YData pos2]);
    |         
    |     end
    |     
    | end
    | 
    | 
    | end
  function DS_updateTraceEff(numAx,pos4,index,drawLine):
    | function DS_updateTraceEff(numAx,pos4,index,drawLine)
    | 
    | coder.extrinsic('delete');
    | coder.extrinsic('scatter');
    | coder.extrinsic('scatter3');
    | coder.extrinsic('getappdata');
    | coder.extrinsic('setappdata');
    | 
    | if(numAx == 4)
    |  
    |     if drawLine
    |         
    |         %udpate Effectuator figure
    |         ax2 = findobj('Tag','TraceAxes2');
    |         punkt2 = getappdata(ax2,'tracePunkt2');
    |         if ~isempty(punkt2)
    |         delete(punkt2);
    |         end
    |         traceLine2 = getappdata(ax2,'traceLine2');
    |         XData2 = get(traceLine2,'XData');
    |         YData2 = get(traceLine2,'YData');
    |         set(traceLine2,'XData',[XData2 index]);
    |         set(traceLine2,'YData',[YData2 pos4]);
    |         
    |     end
    | 
    | end

== stateflow chart EffectuatorIntegratedWithDemonstrator/PosTracer_v1 ==
  state Create_Plot
    entry:
    startPos = DS_createTracePlot(numAxes);
  state Update_Plot
    entry:
    if numAxes == 2
    DS_updateTracePlot(numAxes,pos_x+startPos(1,1),pos_y+startPos(1,2),0,0);
    elseif numAxes == 3
    DS_updateTracePlot(numAxes,pos_x+startPos(1,1),pos_y+startPos(1,2),...
    pos_z+startPos(1,3),0);
    elseif numAxes == 4
    DS_updateTracePlot(numAxes,pos_x+startPos(1,1),pos_y+startPos(1,2),...
    pos_z+startPos(1,3), pos_x2+startPos(1,4));
    end
  state Idle
    during:
    if numAxes == 2
    pos_x = GET_istPos(1);
    pos_y = GET_istPos(2);
    if pos_x ~= old_pos_x
    send(updated_pos);
    end
    if pos_y ~= old_pos_y
    send(updated_pos);
    end
    old_pos_x = pos_x;
    old_pos_y = pos_y;
    elseif numAxes == 3
    pos_x = GET_istPos(1);
    pos_y = GET_istPos(2);
    pos_z = GET_istPos(3);
    if pos_x ~= old_pos_x
    send(updated_pos);
    end
    if pos_y ~= old_pos_y
    send(updated_pos);
    end
    if pos_z ~= old_pos_z
    send(updated_pos);
    end
    elseif numAxes == 4
    pos_x = GET_istPos(1);
    pos_y = GET_istPos(2);
    pos_z = GET_istPos(3);
    pos_x2 = GET_istPos(4);
    if pos_x ~= old_pos_x
    send(updated_pos);
    end
    if pos_y ~= old_pos_y
    send(updated_pos);
    end
    if pos_z ~= old_pos_z
    send(updated_pos);
    end
    if pos_x2 ~= old_pos_x2
    send(updated_pos);
    end
    old_pos_x = pos_x;
    old_pos_y = pos_y;
    old_pos_z = pos_z;
    old_pos_x2 = pos_x2;
    end
  (default) -> Create_Plot
  Create_Plot -> Idle
  Idle -> Update_Plot : updated_pos ...
      | {old_pos_x = pos_x; ...
      | old_pos_y = pos_y; ...
      | old_pos_z = pos_z;...
      | old_pos_x2 = pos_x2}
  Update_Plot -> Idle : after(50,tick)
  data: numAx function_input; sPos function_output; numAx function_input; pos1 function_input; pos2 function_input; pos3 function_input; pos4 function_input; numAxes parameter; pos_x local =0; pos_y local =0; GET_istPos data_store_memory; pos_z local =0; old_pos_x local =0; old_pos_y local =0; old_pos_z local =0; startPos local size=[1 numAxes] =zeros(1,numAxes); pos_x2 local; pold_pos_x2 local
  events: updated_pos local FUNCTION_CALL_EVENT
  function sPos  = DS_createTracePlot(numAx):
    | function sPos  = DS_createTracePlot(numAx)
    | 
    | coder.extrinsic('evalin');
    | 
    | setP = evalin('base','setP_mat');
    | 
    | sPos = zeros(1,numAx);
    | 
    | [~,dim2,~] = size(setP);
    | if(numAx == 3)
    |     fig = figure;
    |     ax = axes;
    |         
    |     
    |     plot3(ax,setP(1,1:dim2),setP(2,1:dim2),setP(3,1:dim2));
    |     
    |     set(fig,'Tag','TraceFig');
    |     set(ax,'Tag','TraceAxes');
    |     set(ax,'NextPlot','add');
    |     
    |     sPos(1,1) = setP(1,1);
    |     sPos(1,2) = setP(2,1);
    |     sPos(1,3) = setP(3,1);
    | elseif (numAx == 4) 
    |     fig = figure;
    |     ax = axes;
    |         
    |     [~,dim2,~] = size(setP);
    |     plot3(ax,setP(1,1:dim2),setP(2,1:dim2),setP(3,1:dim2));
    |     
    |     set(fig,'Tag','TraceFig');
    |     set(ax,'Tag','TraceAxes');
    |     set(ax,'NextPlot','add');
    |     
    |     sPos(1,1) = setP(1,1);
    |     sPos(1,2) = setP(2,1);
    |     sPos(1,3) = setP(3,1);
    |     
    |     %Effectuator axis
    |     fig2 = figure;
    |     ax2 = 1:dim2;
    |     plot(ax2,setP(1,1:dim2));
    |     set(fig2,'Tag','TraceFig');
    |     set(fig2,'Tag','TraceAxes');
    |     set(fig2,'NextPlot','add');
    |     sPos(1,4) = setP(1,1);
    | end
    |     
    | end
  function DS_updateTracePlot(numAx,pos1,pos2,pos3,pos4):
    | function DS_updateTracePlot(numAx,pos1,pos2,pos3,pos4)
    | 
    | coder.extrinsic('delete');
    | coder.extrinsic('scatter3');
    | coder.extrinsic('getappdata');
    | coder.extrinsic('setappdata');
    | 
    | ax = findobj('Tag','TraceAxes');
    | 
    | punkt = getappdata(ax,'tracePunkt');
    | 
    | if ~isempty(punkt)
    |     delete(punkt);
    | end
    | 
    | 
    | if(numAx == 3)
    |    punkt = scatter3(ax,pos1,pos2,pos3,'MarkerEdgeColor','r','LineWidth',2);
    |    setappdata(ax,'tracePunkt',punkt);
    |    
    | elseif(numAx == 4)  
    |    punkt = scatter3(ax,pos1,pos2,pos3,'MarkerEdgeColor','r','LineWidth',2);
    |    setappdata(ax,'tracePunkt',punkt);  
    | end
    | 
    | 
    | end

== stateflow chart EffectuatorIntegratedWithDemonstrator/Joystick Ctrl/Fetch_Global_Data/Chart ==
  state LeseVelOverride
    during:
    vel_x = abs(GET_velocity(1) / (10 * 0.8));
    vel_y = abs(GET_velocity(2) / (5 * 0.8));
    vel_z = abs(GET_velocity(3) / (2 * 0.8));
    velOR_x = VelOverride(1);
    velOR_y = VelOverride(2);
    velOR_z = VelOverride(3);
  (default) -> LeseVelOverride
  data: velOR_x output; velOR_y output; velOR_z output; VelOverride data_store_memory; GET_velocity data_store_memory; vel_x output; vel_y output; vel_z output

== matlab function EffectuatorIntegratedWithDemonstrator/udp_communication/MATLAB Function ==
  data: output output int32; massageSent output int32; setPoints input int32; kooVec input int32; input input int32; massageReceived output int32
function [output,massageSent,massageReceived] = fcn(setPoints,kooVec,input)
% %% Bahnkurve
% 
% setPoints(1,:) = [230,190,110,70,110,190,linspace(230,725,10),230];
% setPoints(2,:) = [75,5,5,75,145,145,75,linspace(75,75,10)];
% setPoints(3,:) = [4,4,0,0,0,4,4,3,2,1,0,0,1,2,3,4,4];
% 
% % Koordinationsmatrix
% 
% kooVec(1,:) = [0,0,0,0,0,0,0,8,11,11,11,11,0,0,0,0];
% kooVec(2,:) = [7,7,7,7,3,3,3,3,7,7,7,7,3,3,3,3];
% kooVec(3,:) = [7,7,7,7,3,3,3,3,12,12,7,7,3,3,3,3];
% kooVec(4,:) = [8,88,8,7,3,3,3,3,7,7,7,7,3,3,3,3];
% kooVec(5,:) = [7,7,7,7,3,3,3,3,7,7,7,7,3,3,6,6];

%% UDP Send Bahnkurve get Koordinationsvektor

massageSent=int32(1);
output=int32(zeros(83,1));
[dataDimZ,dataDimS] = size(setPoints);
output(1:dataDimZ*dataDimS+3,1) = [int32(massageSent);int32(dataDimZ);int32(dataDimS);int32(setPoints(:))];
output(dataDimZ*dataDimS+4:end,1)=int32(0);
massageReceived = input(1);
dataDim1 =[input(2),input(3)];
dataReceived1 = input(4:end);
%koordinationsvektor = int32(reshape(dataReceived1,dataDim1));
koordinationsvektor=int32(dataReceived1);
% UDP Send Koordinationsmatrix get Achse bereit
massageSent=int32(2);
[dataDimZ,dataDimS] = size(kooVec);
output = [massageSent;dataDimZ;dataDimS;kooVec(:)];

massageReceived = input(1);
dataDim2 =[input(2),input(3)];
dataReceived2 = input(4:end);
%Achse_bereit = int32(reshape(dataReceived2,dataDim2));
Achse_bereit=int32(dataReceived2);
% UDP Send Achse start get Achse fertig
massageSent=int32(3);
output(1:3,1) = [int32(massageSent);int32(0);int32(0)];
output(4:end,1)=int32(0);
%pause(0.3);

massageReceived = input(1);
dataDim3 =[input(2),input(3)];
 dataReceived3 = input(4:end);
% Achse_fertig = int32(reshape(dataReceived3,dataDim3));
Achse_fertig=int32(dataReceived3);

== matlab function EffectuatorIntegratedWithDemonstrator/udp_communication/Communication stack/MATLAB Function 5 ==
  data: output1 input int32; output1_isReady input int32; output output int32; output2 input int32; output2_isReady input int32; output3 input int32; output3_isReady input int32; output4 input; output4_isReady input
function output = fcn(output1,output1_isReady,output2,output2_isReady,output3,output3_isReady,output4,output4_isReady)
output = int32(zeros(943,1));
if (output1_isReady==1)
  output=output1;
elseif(output2_isReady==1)
  output=output2;
elseif (output3_isReady==1)
  output=output3; 
elseif (output4_isReady==1)
  output=output4; 
end

== matlab function EffectuatorIntegratedWithDemonstrator/udp_communication/Communication stack/MATLAB Function 1  ==
  settings: sampleTime=Ts
  data: prev_koordinationsvektor input int32; koordinationsvektor output; setPoints input int32; output output int32; massageReceived input; dataDim input int32; dataReceived input; readyToSend output int32; messageFromDispat input int32 size=[1 1]
%function [koordinationsvektor,output,readyToSend]  = fcn(setPoints,massageReceived,dataDim,dataReceived)
function [koordinationsvektor,output,readyToSend]  = fcn(prev_koordinationsvektor,setPoints,massageReceived,dataDim,dataReceived,messageFromDispat)
%% UDP Send Bahnkurve get Koordinationsvektor
output=int32(zeros(943,1));
if(massageReceived==0&&messageFromDispat==0)
massageSent=int32(1);
[dataDimZ,dataDimS] = size(setPoints);
output(1:dataDimZ*dataDimS+3,1) = [int32(massageSent);int32(dataDimZ);int32(dataDimS);int32(setPoints(:))];
output(dataDimZ*dataDimS+4:end,1)=int32(0);
readyToSend=int32(1);
else
readyToSend=int32(0);
end
 if(massageReceived==1)
 koordinationsvektor=int32(dataReceived);
 else
 koordinationsvektor=prev_koordinationsvektor;
 end

== matlab function EffectuatorIntegratedWithDemonstrator/udp_communication/Communication stack/MATLAB Function 3 ==
  data: Achse_fertig output int32; output output int32; massageReceived input int32; dataDim input int32; dataReceived input int32; readyToSend output int32; messageFromDispat input
    function [Achse_fertig,output,readyToSend]  = fcn(massageReceived,dataDim,dataReceived,messageFromDispat)
% UDP Send Achse start get Achse fertig
output=int32(zeros(943,1));
if(massageReceived==2&&messageFromDispat==2)
massageSent=int32(3);
output(1:3,1) = [int32(massageSent);int32(0);int32(0)];
output(4:end)=0;
readyToSend=int32(1);
else
readyToSend=int32(0);
end
 if(massageReceived==4)
 Achse_fertig=int32(1);
 else
 Achse_fertig=int32(0);
 end

== matlab function EffectuatorIntegratedWithDemonstrator/udp_communication/Communication stack/MATLAB Function 4 ==
  data: prev_EffSegmentData input; EffSegmentData output int32; output output int32; massageReceived input int32; dataDim input int32; dataReceived input int32; readyToSend output int32; axesPos input
function [EffSegmentData,output,readyToSend]  = fcn(prev_EffSegmentData,massageReceived,dataDim,dataReceived,axesPos)
% UDP Send axes postion
output=int32(zeros(943,1));
if(massageReceived==3)
massageSent=int32(4);
output(1:7,1) = [int32(massageSent);int32(1);int32(4);axesPos];
output(11:end)=0;
readyToSend=int32(1);
EffSegmentData=dataReceived(1:3);
else
readyToSend=int32(0);
EffSegmentData=prev_EffSegmentData;
end

== matlab function EffectuatorIntegratedWithDemonstrator/udp_communication/UDP Send//Receive/udp_receive/MATLAB Function ==
  data: input input int32; massageReceived output int32; dataDim output int32; dataReceived output int32
function [massageReceived,dataDim,dataReceived] = fcn(input)
massageReceived = input(1);
dataDim =[input(2),input(3)];
dataReceived = (input(4:end))';

== matlab function EffectuatorIntegratedWithDemonstrator/udp_communication/Communication stack/MATLAB Function 2 ==
  data: prev_Achse_bereit input int32; Achse_bereit output int32; kooVec input int32; output output int32; massageReceived input int32; dataDim input int32; dataReceived input int32; readyToSend output int32; messageFromDispat input int32
function [Achse_bereit,output,readyToSend]   = fcn(prev_Achse_bereit,kooVec,massageReceived,dataDim,dataReceived,messageFromDispat)
% UDP Send Koordinationsmatrix get Achse bereit
output=int32(zeros(943,1));
if (massageReceived==1&&messageFromDispat==1)
massageSent=int32(2);
[dataDimZ,dataDimS] = size(kooVec);
output(1:dataDimZ*dataDimS+3,1) = [massageSent;dataDimZ;dataDimS;kooVec(:)];
output(dataDimZ*dataDimS+4:end,1)=0;
readyToSend=int32(1);
else
readyToSend=int32(0);
end
 if (massageReceived==2)
 Achse_bereit=int32(dataReceived);
 else
 Achse_bereit=prev_Achse_bereit;    
 end

== matlab function EffectuatorIntegratedWithDemonstrator/MATLAB Function ==
  data: x input; y input; z input; output output; s_index input
function output = fcn(x,y,z,s_index)
output=[x;y;z;s_index]
